simulink subsystem "TOFs"  (R2024b)
settings: Solver=VariableStepAuto  StartTime=0.0  StopTime=10.0  RelTol=1e-3
undefined symbols (not defined in the file or in its folder): samplingTime
settings Model: Creator=JesseJabezArendse  LastModifiedBy=JesseJabezArendse

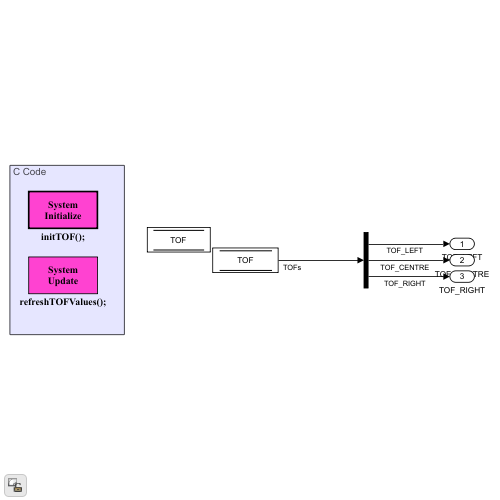
[thumbnail: Simulink's stored preview of the top-level diagram]
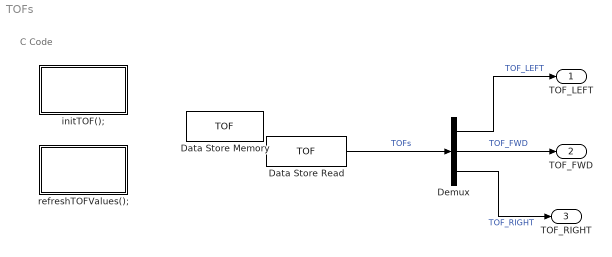
== system TOFs ==
  note: C Code
  Data Store Memory : DataStoreMemory  DataStoreName=TOF  WriteAfterWriteMsg=warning  ShowAdditionalParam=off  OutDataTypeStr=single  Dimensions=3
  Data Store Read : DataStoreRead  DataStoreName=TOF  IndexOptions=Index vector (dialog)  Indices=1  OutputSizes=1
  Demux : Demux  Outputs=3
  initTOF(); : Subsystem  TreatAsAtomicUnit=on  SystemSampleTime=samplingTime  mask(System Initialize){ShowInLibBrowser=0}
      mask prompts: ShowInLibBrowser "Simulink:masks:CustCodeMaskParam1_MP"
      settings: CopyFcn=cccopyfcn(gcb)  OpenFcn=ccopenfcn('System Initialize Function')
      mask Help: eval('feval(''rtwprivate'',''rtwhelpview'',''rtw_sys_initialize_block'')');
      mask DialogControl ShowInLibBrowser Prompt: Mask Parameter 1:
      mask Display: disp('System\nInitialize');
  refreshTOFValues(); : Subsystem  mask(System Update){ShowInLibBrowser=0}
      mask prompts: ShowInLibBrowser "Simulink:masks:CustCodeMaskParam1_MP"
      settings: CopyFcn=cccopyfcn(gcb)  OpenFcn=ccopenfcn('System Update Function')
      mask Help: eval('feval(''rtwprivate'',''rtwhelpview'',''rtw_sys_update_block'')');
      mask Display: disp('System\nUpdate');
  TOF_LEFT : Outport
  TOF_FWD : Outport  Port=2
  TOF_RIGHT : Outport  Port=3
  wires:
  Demux/1 -> TOF_LEFT/1  "TOF_LEFT"
  Data Store Read/1 -> Demux/1  "TOFs"
  Demux/2 -> TOF_FWD/1  "TOF_FWD"
  Demux/3 -> TOF_RIGHT/1  "TOF_RIGHT"

== system TOFs/initTOF(); ==

== system TOFs/refreshTOFValues(); ==
